simulink model "Hw1_2_b"  (R2015b)
settings: Solver=VariableStepAuto  StartTime=0.0  StopTime=25  RelTol=1e-3
settings Model: Creator=user  LastModifiedBy=user

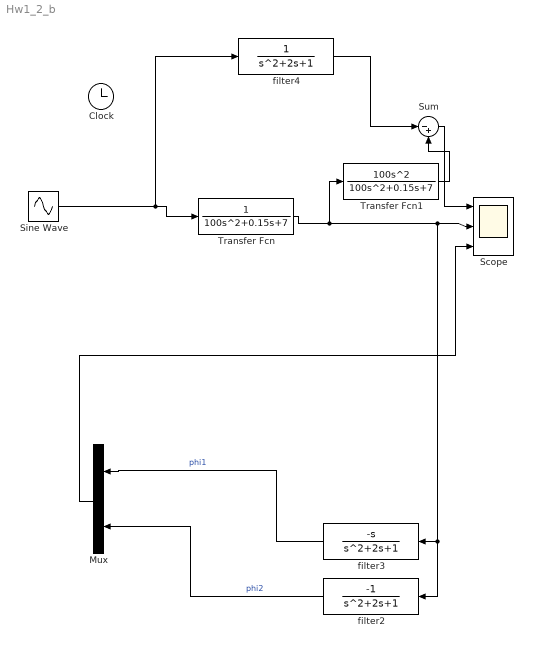
== system Hw1_2_b ==
  Clock : Clock
      settings: Decimation=250
  Mux : Mux  Inputs=2
  Scope : Scope  NumInputPorts=3
  Sine Wave : Sin  Bias=1  Frequency=pi/3  Phase=pi/2  SampleTime=0
  Sum : Sum  Inputs=|-+
  Transfer Fcn : TransferFcn  Denominator=[100 0.15 7]
  Transfer Fcn1 : TransferFcn  Numerator=[100 0 0]  Denominator=[100 0.15 7]
  filter2 : TransferFcn  Numerator=[-1 ]
  filter3 : TransferFcn  Numerator="[-1  0]"
  filter4 : TransferFcn
  wires:
  Sine Wave/1 -> filter4/1, Transfer Fcn/1
  Transfer Fcn/1 -> Transfer Fcn1/1, filter2/1, filter3/1, Scope/2
  filter3/1 -> Mux/1  "phi1"
  filter2/1 -> Mux/2  "phi2"
  Mux/1 -> Scope/3
  filter4/1 -> Sum/1
  Transfer Fcn1/1 -> Sum/2
  Sum/1 -> Scope/1
